simulink model "normalization3"  (R2023b)
settings: Solver=VariableStepAuto  StartTime=0.0  StopTime=30  RelTol=1e-3
PreLoadFcn:
  | buffer_tiling
InitFcn:
  | buffer_tiling
values from neighbouring files (symbols this model uses):
  COL = 256    [run_model.m]    (also in setup.m)
  mtxA_r = [mtxA_r, pattern]    [buffer_tiling.m]
  mtxA_w = [mtxA_w, pattern]    [buffer_tiling.m]
  mtxB_r = [mtxB_r, pattern]    [buffer_tiling.m]
  mtxB_w = [mtxB_w, pattern]    [buffer_tiling.m]
  PLIO_NUM = 3    [run_model.m]    (also in setup.m)
  ROW = 384    [run_model.m]    (also in setup.m)
undefined symbols (not defined in the file or in its folder): AIE, ML, S, vsvh1760, xcve2802
libraries: aieUtilities x9, dspstat3 x2, aieBasic x2, vmcUtilities x1
settings Model: Creator=robg  LastModifiedBy=abehbood
settings DataIOCC: ReturnWorkspaceOutputs=off
settings OptimizationCC: ReuseModelBlockBuffer=off
settings SFSimCC: SimTargetLang=C++

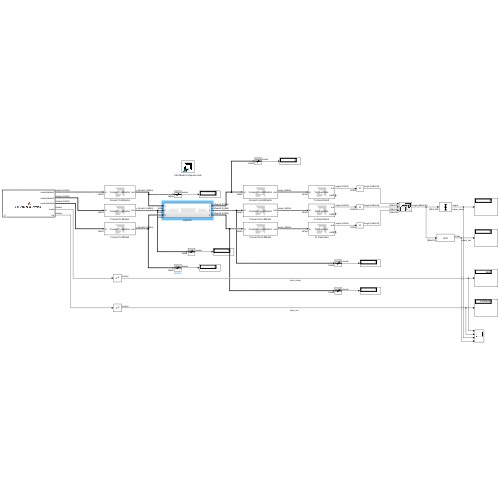
[thumbnail: Simulink's stored preview of the top-level diagram]
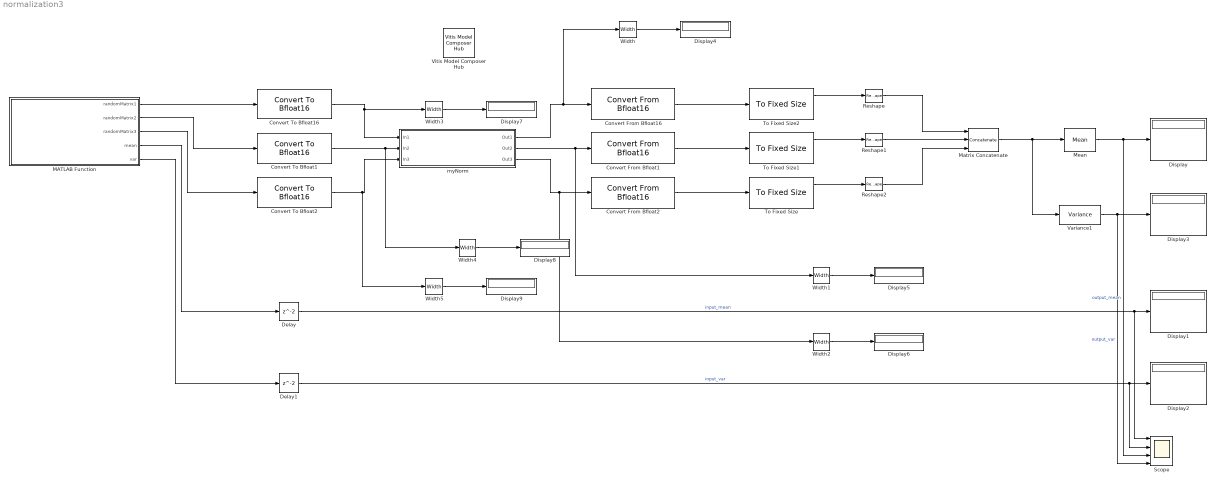
== system normalization3 ==
  Convert From Bfloat1 : aieUtilities/Convert From Bfloat16  OutputDataType=single
  Convert From Bfloat16 : aieUtilities/Convert From Bfloat16  OutputDataType=single
  Convert From Bfloat2 : aieUtilities/Convert From Bfloat16  OutputDataType=single
  Convert To Bfloat1 : aieUtilities/Convert To Bfloat16
  Convert To Bfloat16 : aieUtilities/Convert To Bfloat16
  Convert To Bfloat2 : aieUtilities/Convert To Bfloat16
  Delay : Delay
  Delay1 : Delay
  Display{,1..9} (10 alike) : Display
  MATLAB Function : MATLAB Function  TreatAsAtomicUnit=on  mask{numRows=ROW, numCols=COL}
      mask prompts: numRows "Number of Rows"; numCols "Number of  Columns"
  Matrix Concatenate : Concatenate  NumInputs=3  Mode=Multidimensional array
  Mean : dspstat3/Mean  run=off  InputProcessing=Columns as channels (frame based)  reset_popup=None  directionMode=Entire input  dimension=1  roiEnable=off  roiType=Rectangles  roiPortion=Entire ROI  roiOutput=Individual statistics for each ROI  roiFlag=off  roundingMode=Floor  overflowMode=off  outputDataTypeStr=Inherit: Same as accumulator  outputMin=[]  outputMax=[]  outputLastDataTypeStr=Inherit: Same as accumulator
  Reshape : Reshape  OutputDimensionality=Customize  OutputDimensions=[ROW/PLIO_NUM,COL]
  Reshape1 : Reshape  OutputDimensionality=Customize  OutputDimensions=[ROW/PLIO_NUM,COL]
  Reshape2 : Reshape  OutputDimensionality=Customize  OutputDimensions=[ROW/PLIO_NUM,COL]
  Scope : Scope  NumInputPorts=4
  To Fixed Size : aieUtilities/To Fixed Size  Mode=Produce a valid output signal  OutputSize=Inherit: Same as input  CopyMethod=Buffer samples to form output  HasStatusOutput=on
  To Fixed Size1 : aieUtilities/To Fixed Size  Mode=Produce a valid output signal  OutputSize=Inherit: Same as input  CopyMethod=Buffer samples to form output  HasStatusOutput=on
  To Fixed Size2 : aieUtilities/To Fixed Size  Mode=Produce a valid output signal  OutputSize=Inherit: Same as input  CopyMethod=Buffer samples to form output  HasStatusOutput=on
  Variance1 : dspstat3/Variance  run=off  InputProcessing=Columns as channels (frame based)  reset_popup=None  directionMode=Entire input  dimension=1  roiEnable=off  roiType=Rectangles  roiPortion=Entire ROI  roiOutput=Individual statistics for each ROI  roiFlag=off  roundingMode=Floor  overflowMode=off
  Vitis Model Composer Hub : vmcUtilities/Vitis Model Composer Hub  Tag=genX  CodeGeneration=off  SubsystemName=myNorm  CompilationType=AIECompilation  SubsystemType=AIENode  ExportTypeV2=Graph Code  TargetDirectory=./code  exportDesign=off  analyzeDesign=on  validateDesignOnHw=off  ExportType=AI Engines  IpVendor=xilinx.com  IpLibrary=hls  IpVersion=1.0  IpHWLanguage=Verilog  AieCompilerOptions={}  AieSimulatorOptions={}  CreateTestbench=on  TestbenchStackSize=10  RunRtlSim=off  RunCSim=off  RunAieSim=on  AieSimTimeout=50000  RunAieSimProfiling=off  LaunchVitisAnalyzer=off  PlotOutput=off  RunX86Sim=off  X86SimTimeout=10  GenHwImage=off  GenLibadfXo=off  GenHwValidationCode=off  PlatformType=Specify Platform  Platform=/proj/xbuilds/SWIP/2024.1_0414_2055/installs/lin64/Vitis/2024.1/base_platforms/xilinx_vek280_base_202410_1/xilinx_vek280_base_202410_1.xpfm  HwSystemType=Baremetal  HwValidationTarget=hw_emu  ProjDevice=Versal VEK280 Evaluation Platform with FMC Connector (xcve2802-vsvh1760-2MP-e-S)  ProjDevicePart=xcve2802-vsvh1760-2MP-e-S  AIEType=AIE-ML  SamplePeriod=-1  ClockFrequency=200  DataPathParallelism=1  xilinxfamily=versalaiedge  part=xcve2802  speed=-2MP-e-S  package=vsvh1760  directory=./netlist  testbench=off  incr_netlist=off  synthesis_tool=Vivado  clock_wrapper=Clock Enables  dbl_ovrd=According to Block Masks  dcm_input_clock_period=10  sysclk_period=10  simulink_period=1  eval_field=0  IPInfoJsonString="{\"AIESubsystem\":{\"SubsystemName\":\"myNorm\",\"TargetDirectory\":\"./code\",\"SubsystemDir\":\"./code/ip/myNorm\"},\"SubsystemTag\":\"AIENode\"}"  LogFileName=/proj/xsjhdstaff4/abehbood/vmc_examples/gitent_ws/Examples/AIENGINE/Normalization/code/model_composer.log  NThreads=4
  Width{,1..5} (6 alike) : Width
  myNorm : Subsystem
  wires:
  myNorm/2(Out2) -> Width1/1, Convert From Bfloat1/1
  myNorm/3(Out3) -> Convert From Bfloat2/1, Width2/1
  Convert From Bfloat16/1 -> To Fixed Size2/1
  To Fixed Size2/1 -> Reshape/1
  To Fixed Size1/1 -> Reshape1/1
  To Fixed Size/1 -> Reshape2/1
  Reshape/1 -> Matrix Concatenate/1
  Reshape1/1 -> Matrix Concatenate/2
  Reshape2/1 -> Matrix Concatenate/3
  Matrix Concatenate/1 -> Variance1/1, Mean/1
  Mean/1 -> Scope/3, Display/1  "output_mean"
  MATLAB Function/5(var) -> Delay1/1
  Variance1/1 -> Scope/4, Display3/1  "output_var"
  MATLAB Function/4(mean) -> Delay/1
  MATLAB Function/1(randomMatrix1) -> Convert To Bfloat16/1
  MATLAB Function/2(randomMatrix2) -> Convert To Bfloat1/1
  MATLAB Function/3(randomMatrix3) -> Convert To Bfloat2/1
  Convert To Bfloat16/1 -> Width3/1, myNorm/1(In1)
  Convert To Bfloat1/1 -> Width4/1, myNorm/2(In2)
  Convert To Bfloat2/1 -> Width5/1, myNorm/3(In3)
  Delay/1 -> Scope/1, Display1/1  "input_mean"
  Delay1/1 -> Scope/2, Display2/1  "input_var"
  Convert From Bfloat2/1 -> To Fixed Size/1
  Width1/1 -> Display5/1
  Convert From Bfloat1/1 -> To Fixed Size1/1
  Width2/1 -> Display6/1
  Width3/1 -> Display7/1
  Width4/1 -> Display8/1
  Width5/1 -> Display9/1
  myNorm/1(Out1) -> Width/1, Convert From Bfloat16/1
  Width/1 -> Display4/1

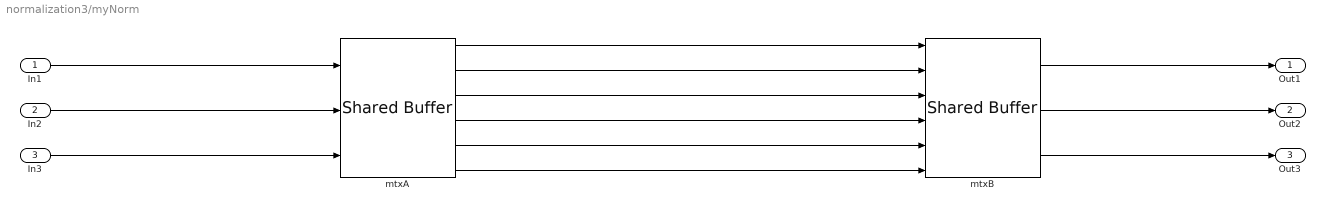
== system normalization3/myNorm ==
  In1 : Inport
  In2 : Inport  Port=2
  In3 : Inport  Port=3
  mtxA : aieBasic/Shared Buffer  DataType=bfloat16  NumBuffer=1  BufferDim=[ROW,COL]  NumInput=3  NumOutput=6  RepetitionCount=0  Input0Tiling=mtxA_w(1)  Input1Tiling=mtxA_w(2)  Input2Tiling=mtxA_w(3)  Input3Tiling=[]  Input4Tiling=[]  Input5Tiling=[]  Output0Tiling=mtxA_r(1)  Output1Tiling=mtxA_r(2)  Output2Tiling=mtxA_r(3)  Output3Tiling=mtxA_r(4)  Output4Tiling=mtxA_r(5)  Output5Tiling=mtxA_r(6)  InBuffDims={128, 384}|{128, 384}|{128, 384}  InTilingDims={128, 128}|{128, 128}|{128, 128}  InOffsets={0, 0}|{0, 128}|{0, 256}  InTileTraveseDims={}|{}|{}  InTileTraveseStrides={}|{}|{}  InTileTraveseWraps={}|{}|{}  InPacketPortIDs={}|{}|{}  InRepetitions={}|{}|{}  InBoundaryDims={}|{}|{}  OutBuffDims={128, 384}|{128, 384}|{128, 384}|{128, 384}|{128, 384}|{128, 384}  OutTilingDims={128, 64}|{128, 64}|{128, 64}|{128, 64}|{128, 64}|{128, 64}  OutOffsets={0, 0}|{0, 64}|{0, 128}|{0, 192}|{0, 256}|{0, 320}  OutTileTraveseDims={}|{}|{}|{}|{}|{}  OutTileTraveseStrides={}|{}|{}|{}|{}|{}  OutTileTraveseWraps={}|{}|{}|{}|{}|{}  OutPacketPortIDs={}|{}|{}|{}|{}|{}  OutRepetitions={}|{}|{}|{}|{}|{}  OutBoundaryDims={}|{}|{}|{}|{}|{}  BufferDimStr={384, 128}  blockJsonConstraints=[]  deprecateConstraints=0
  mtxB : aieBasic/Shared Buffer  DataType=bfloat16  NumBuffer=1  BufferDim=[COL,ROW]  NumInput=6  NumOutput=3  RepetitionCount=0  Input0Tiling=mtxB_w(1)  Input1Tiling=mtxB_w(2)  Input2Tiling=mtxB_w(3)  Input3Tiling=mtxB_w(4)  Input4Tiling=mtxB_w(5)  Input5Tiling=mtxB_w(6)  Output0Tiling=mtxB_r(1)  Output1Tiling=mtxB_r(2)  Output2Tiling=mtxB_r(3)  Output3Tiling=struct('buffer_dimension', [256,384], 'tiling_dimension', [256,64], 'offset', [0,64*3])  Output4Tiling=struct('buffer_dimension', [256,384], 'tiling_dimension', [256,64], 'offset', [0,64*4])  Output5Tiling=struct('buffer_dimension', [256,384], 'tiling_dimension', [256,64], 'offset', [0,64*5])  InBuffDims={128, 384}|{128, 384}|{128, 384}|{128, 384}|{128, 384}|{128, 384}  InTilingDims={128, 64}|{128, 64}|{128, 64}|{128, 64}|{128, 64}|{128, 64}  InOffsets={0, 0}|{0, 64}|{0, 128}|{0, 192}|{0, 256}|{0, 320}  InTileTraveseDims={}|{}|{}|{}|{}|{}  InTileTraveseStrides={}|{}|{}|{}|{}|{}  InTileTraveseWraps={}|{}|{}|{}|{}|{}  InPacketPortIDs={}|{}|{}|{}|{}|{}  InRepetitions={}|{}|{}|{}|{}|{}  InBoundaryDims={}|{}|{}|{}|{}|{}  OutBuffDims={128, 384}|{128, 384}|{128, 384}  OutTilingDims={128, 128}|{128, 128}|{128, 128}  OutOffsets={0, 0}|{0, 128}|{0, 256}  OutTileTraveseDims={}|{}|{}  OutTileTraveseStrides={}|{}|{}  OutTileTraveseWraps={}|{}|{}  OutPacketPortIDs={}|{}|{}  OutRepetitions={}|{}|{}  OutBoundaryDims={}|{}|{}  BufferDimStr={128, 384}  blockJsonConstraints=[]  deprecateConstraints=0
  Out1 : Outport
  Out2 : Outport  Port=2
  Out3 : Outport  Port=3
  wires:
  mtxB/3 -> Out3/1
  In3/1 -> mtxA/3
  mtxB/1 -> Out1/1
  mtxB/2 -> Out2/1
  In1/1 -> mtxA/1
  In2/1 -> mtxA/2
  mtxA/1 -> mtxB/1
  mtxA/2 -> mtxB/2
  mtxA/3 -> mtxB/3
  mtxA/4 -> mtxB/4
  mtxA/5 -> mtxB/5
  mtxA/6 -> mtxB/6

== matlab function normalization3/MATLAB Function ==
  settings: updateMethod=DISCRETE  sampleTime=1
  data: randomMatrix1 output size=ROW*COL/3; numRows parameter; numCols parameter; randomMatrix2 output size=ROW*COL/3; randomMatrix3 output size=ROW*COL/3; mean output; var output
function [randomMatrix1, randomMatrix2, randomMatrix3, mean, var] = generateRandomMatrix(numRows, numCols)

persistent p 

if isempty(p)
    p = 0;
end

randomMean = rand(1)*2^14+128;
randomGain = rand(1)*2^14+128;

if rem(p,3)==0
    randomMatrix = randn(numRows*numCols,1)*randomGain + randomMean; % Generate random matrix

    randomMatrix1 = randomMatrix(1:numRows/3*numCols);
    randomMatrix2 = randomMatrix(numRows/3*numCols+1:numRows*2/3*numCols);
    randomMatrix3 = randomMatrix(numRows*2/3*numCols+1:end);
    mean = randomMean;
    var = randomGain.^2;

else
    randomMatrix1 = [];
    randomMatrix2 = [];
    randomMatrix3 = [];
    mean = 0;
    var = 0;
end


p = p+1;
